simulink model "pdl_nonlinear_hw2"  (R2017a)
settings: Solver=VariableStepAuto  StartTime=0.0  StopTime=duration  RelTol=1e-3
values from neighbouring files (symbols this model uses):
  b = 0.1    [pendulum_hw2.m]
  f_p = 1e-4    (= 0.0001)    [pendulum_hw2.m]
  g = 9.81    [pendulum_hw2.m]
  K = lqr(A,B,Q,R)    [pendulum_hw2.m]
  k = 0.15    [pendulum_hw2.m]
  L = 1.4    [pendulum_hw2.m]
  m = 0.75    [pendulum_hw2.m]
  M = 1    [pendulum_hw2.m]
  m_p = 1e-7    (= 1e-07)    [pendulum_hw2.m]
  Nbar = -pinv(B)*A*pinv(Cn)+K*pinv(Cn)    [pendulum_hw2.m]
  Ts = 0.001    [pendulum_hw2.m]
  w_p = 10    [pendulum_hw2.m]
libraries: simulink x3, simulink_extras x2
settings Model: Creator=Salmon  LastModifiedBy=Salmon

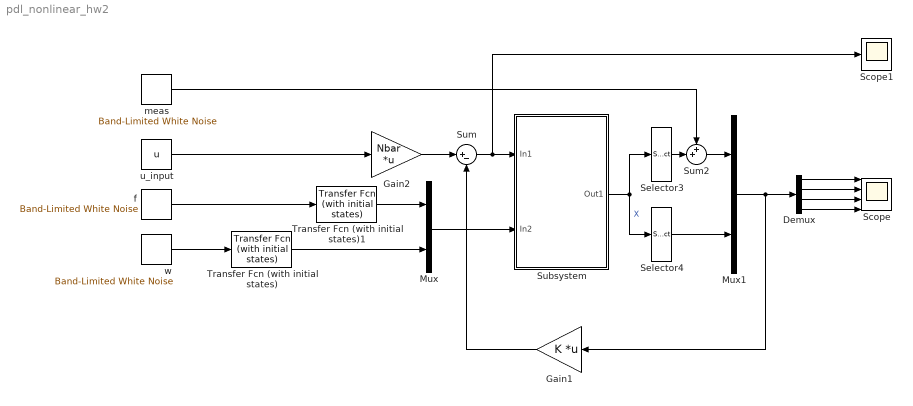
== system pdl_nonlinear_hw2 ==
  Demux : Demux
  Gain1 : Gain  Gain=K  Multiplication=Matrix(K*u)
  Gain2 : Gain  Gain=Nbar  Multiplication=Matrix(K*u)
  Mux : Mux  Inputs=2
  Mux1 : Mux  Inputs=2
  Scope : Scope  NumInputPorts=4
  Scope1 : Scope
  Selector3 : Selector  InputPortWidth=4  IndexOptions=Index vector (dialog)  Indices=[1 2]  OutputSizes=1
  Selector4 : Selector  InputPortWidth=4  IndexOptions=Index vector (dialog)  Indices=[3 4]  OutputSizes=1
  Subsystem : Subsystem
  Sum : Sum  Inputs=|+-
  Sum2 : Sum  Inputs=++|
  Transfer Fcn (with initial states) : simulink_extras/Additional Linear/Transfer Fcn (with initial states)  N=[0.64]  D="[1  0.8]"  X0=0
  Transfer Fcn (with initial states)1 : simulink_extras/Additional Linear/Transfer Fcn (with initial states)  N=[0.64]  D="[1  0.8]"  X0=0
  f : simulink/Sources/Band-Limited White Noise  Cov=[f_p]  Ts=Ts  seed=[23341]
  meas : simulink/Sources/Band-Limited White Noise  Cov=[m_p,m_p]  Ts=Ts  seed=[123,23341]
  u_input : Constant  Value=u
  w : simulink/Sources/Band-Limited White Noise  Cov=[w_p]  Ts=Ts  seed=[23341]
  wires:
  u_input/1 -> Gain2/1
  f/1 -> Transfer Fcn (with initial states)1/1
  w/1 -> Transfer Fcn (with initial states)/1
  Mux/1 -> Subsystem/2(In2)
  Gain1/1 -> Sum/2
  Mux1/1 -> Gain1/1, Demux/1
  Gain2/1 -> Sum/1
  Sum/1 -> Subsystem/1(In1), Scope1/1
  Sum2/1 -> Mux1/1
  Selector4/1 -> Mux1/2
  Selector3/1 -> Sum2/2
  Subsystem/1(Out1) -> Selector4/1, Selector3/1  "X"
  meas/1 -> Sum2/1
  Demux/1 -> Scope/1
  Demux/2 -> Scope/2
  Demux/3 -> Scope/3
  Demux/4 -> Scope/4
  Transfer Fcn (with initial states)1/1 -> Mux/1
  Transfer Fcn (with initial states)/1 -> Mux/2

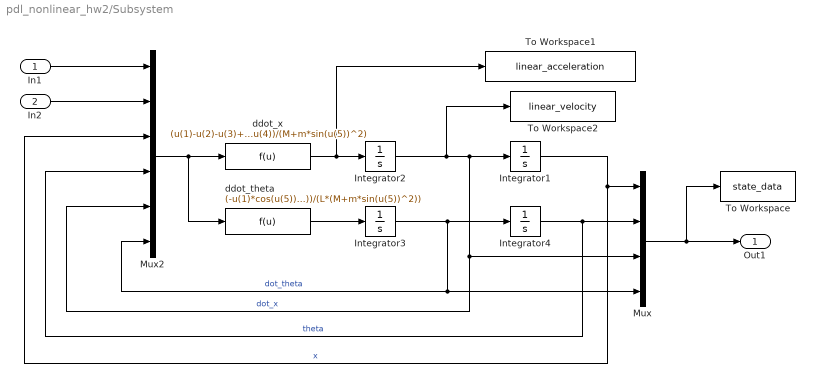
== system pdl_nonlinear_hw2/Subsystem ==
  In1 : Inport
  In2 : Inport  Port=2
  Integrator{1..4} (4 alike) : Integrator
  Mux : Mux
  Mux2 : Mux  Inputs=6
  To Workspace : ToWorkspace  VariableName=state_data  SaveFormat=Structure With Time  SampleTime=-1
  To Workspace1 : ToWorkspace  VariableName=linear_acceleration  SaveFormat=Structure With Time  SampleTime=-1
  To Workspace2 : ToWorkspace  VariableName=linear_velocity  SaveFormat=Structure With Time  SampleTime=-1
  ddot_theta : Fcn  Expr=(-u(1)*cos(u(5))+u(3)*cos(u(5))-m*L*u(7)^2*sin(u(5))*cos(u(5))+(M+m)*g*sin(u(5))-(M/m)*u(2)*cos(u(5))+b*u(6)*cos(u(5))+k*u(4)*cos(u(5)))/(L*(M+m*sin(u(5))^2))
  ddot_x : Fcn  Expr=(u(1)-u(2)-u(3)+u(2)*cos(u(5))^2+m*L*u(7)^2*sin(u(5))-m*g*sin(u(5))*cos(u(5))-b*u(6)-k*u(4))/(M+m*sin(u(5))^2)
  Out1 : Outport
  wires:
  Integrator3/1 -> Mux2/6, Mux/4, Integrator4/1  "dot_theta"
  In2/1 -> Mux2/2
  ddot_x/1 -> To Workspace1/1, Integrator2/1
  Integrator2/1 -> To Workspace2/1, Mux2/5, Mux/3, Integrator1/1  "dot_x"
  ddot_theta/1 -> Integrator3/1
  Mux/1 -> Out1/1, To Workspace/1
  In1/1 -> Mux2/1
  Integrator1/1 -> Mux2/3, Mux/1  "x"
  Mux2/1 -> ddot_theta/1, ddot_x/1
  Integrator4/1 -> Mux2/4, Mux/2  "theta"
